simulink model "IrbotCreateModel"  (R2015a)
settings: Solver=ode45  StartTime=0.0  StopTime=10  RelTol=1e-3
model workspace (MAT data in the model file):
  X0 = [5 6 1.0471975512]
  l = 0.263
  R = 0.1315
libraries: simulink x1
settings Model: Creator=pic  LastModifiedBy=Sean
settings DataIOCC: SignalLoggingSaveFormat=ModelDataLogs
settings OptimizationCC: ExpressionDepthLimit=2147483647
settings DebuggingCC: UnderspecifiedInitializationDetection=Classic  MergeDetectMultiDrivingBlocksExec=none  SolverPrmCheckMsg=warning  FcnCallInpInsideContextMsg=UseLocalSettings  StateNameClashWarn=warning
settings GRTTargetCC: CombineOutputUpdateFcns=off  GRTInterface=on

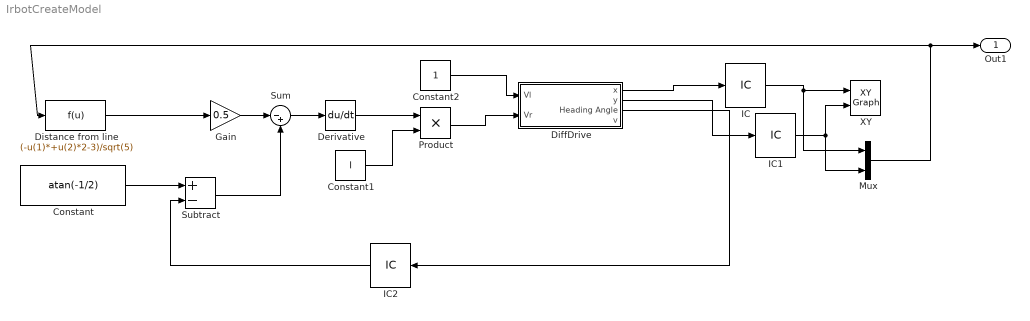
== system IrbotCreateModel ==
  Constant : Constant  Value=atan(-1/2)
  Constant1 : Constant  Value=l
  Constant2 : Constant
  Derivative : Derivative
  "DiffDrive " : Subsystem
  Distance from line : Fcn  Expr=(-u(1)*+u(2)*2-3)/sqrt(5)
  Gain : Gain  Gain=0.5
  IC : InitialCondition  Value=5
  IC1 : InitialCondition  Value=6
  IC2 : InitialCondition  Value=pi/3
  Mux : Mux  Inputs=2
  Product : Product
  Subtract : Sum  Inputs=+-
  Sum : Sum  Inputs=|-+
  XY : simulink/Sinks/XY Graph  xmin=0  xmax=10  ymin=0  ymax=10  st=-1
  Out1 : Outport
  wires:
  "DiffDrive "/3(Heading Angle) -> IC2/1
  "DiffDrive "/1(x) -> IC/1
  "DiffDrive "/2(y) -> IC1/1
  Constant/1 -> Subtract/1
  Mux/1 -> Out1/1, Distance from line/1
  Distance from line/1 -> Gain/1
  Gain/1 -> Sum/1
  Subtract/1 -> Sum/2
  Sum/1 -> Derivative/1
  Derivative/1 -> Product/1
  Product/1 -> "DiffDrive "/2(Vr)
  Constant1/1 -> Product/2
  Constant2/1 -> "DiffDrive "/1(Vl)
  IC2/1 -> Subtract/2
  IC1/1 -> Mux/2, XY/2
  IC/1 -> Mux/1, XY/1

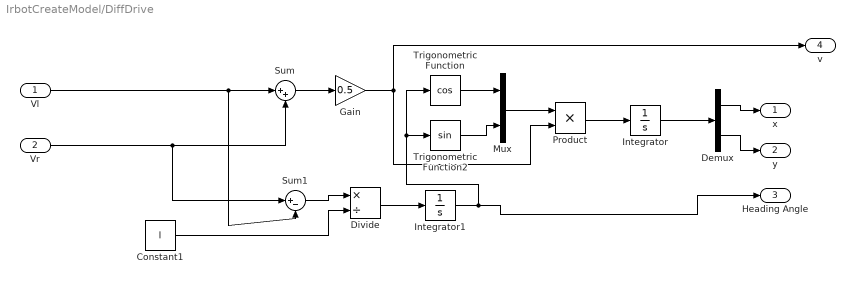
== system IrbotCreateModel/DiffDrive  ==
  Vl : Inport
  Vr : Inport  Port=2
  Constant1 : Constant  Value=l
  Demux : Demux  Outputs=2
  Divide : Product  Inputs=*/
  Gain : Gain  Gain=0.5
  Integrator : Integrator
  Integrator1 : Integrator
  Mux : Mux  Inputs=2
  Product : Product  RndMeth=Zero
  Sum : Sum  Inputs=|++
  Sum1 : Sum  Inputs=|+-
  Trigonometric Function : Trigonometry  Operator=cos
  Trigonometric Function2 : Trigonometry
  x : Outport
  y : Outport  Port=2
  Heading Angle : Outport  Port=3
  v : Outport  Port=4
  wires:
  Trigonometric Function/1 -> Mux/1
  Product/1 -> Integrator/1
  Integrator/1 -> Demux/1
  Demux/1 -> x/1
  Demux/2 -> y/1
  Mux/1 -> Product/1
  Trigonometric Function2/1 -> Mux/2
  Vl/1 -> Sum1/2, Sum/1
  Vr/1 -> Sum/2, Sum1/1
  Sum/1 -> Gain/1
  Sum1/1 -> Divide/1
  Constant1/1 -> Divide/2
  Gain/1 -> Product/2, v/1
  Divide/1 -> Integrator1/1
  Integrator1/1 -> Trigonometric Function2/1, Trigonometric Function/1, Heading Angle/1
